simulink model "inverter_network"  (R2023a)
settings: Solver=ode4  StartTime=0.0  StopTime=0.8  FixedStep=1e-6  RelTol=1e-3
values from neighbouring files (symbols this model uses):
  C_gv = 1.5e-3    (= 0.0015)    [init.m]
  Cf = 2e-5    (= 2e-05)    [init.m]
  Cf_r = 1    [init.m]
  frequency = 50    [init.m]
  kpgi = 15    [init.m]
  kpi = 8    [init.m]
  kpv = 0.1    [init.m]
  krgi = 600    [init.m]
  krv = 100    [init.m]
  L_fv = 1.5e-3    (= 0.0015)    [init.m]
  L_line = 0.003*rbase/omega    (= 0.000152788745368)    [init.m]
  Lf = 4e-3    (= 0.004)    [init.m]
  Lf_r = 0.3    [init.m]
  Lg = 0.24e-3    (= 0.00024)    [init.m]
  omega = 2*pi*frequency    (= 314.159265359)    [init.m]
  R_line = 0.013*rbase    (= 0.208)    [init.m]
  vc_l = 0.03*rbase    (= 0.48)    [init.m]
  vdc = 400*1.88    (= 752)    [init.m]
  vref_rms = 300*(0.707*sqrt(3))    [init.m]
libraries: spsThreePhaseVIMeasurementLib x14, spsHalfBridgeConverterLib x9, spsThreePhaseSeriesRLCBranchLib x7, spsPower3phInstantaneousLib x6, spsThreePhaseParallelRLCBranchLib x5, spsabctoAlphaBetaZeroLib x5, spsGroundLib x4, spsAlphaBetaZerotoabcLib x3, spsDCVoltageSourceLib x3, eePwmGeneratorTwoLevel x3, spsPLL3phLib x2, spsdq0toAlphaBetaZeroLib x2
(part 1 of 2)
settings Model: Creator=MrSam  LastModifiedBy=15185

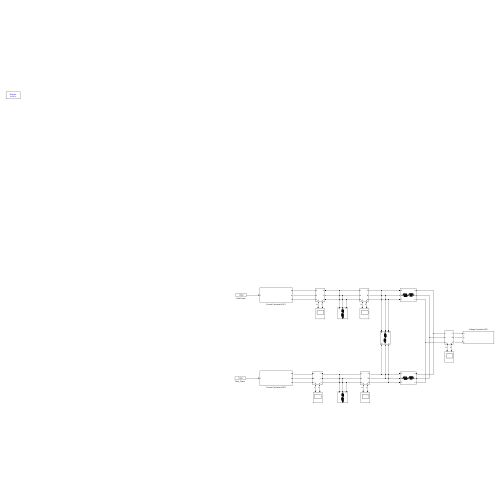
[thumbnail: Simulink's stored preview of the top-level diagram]
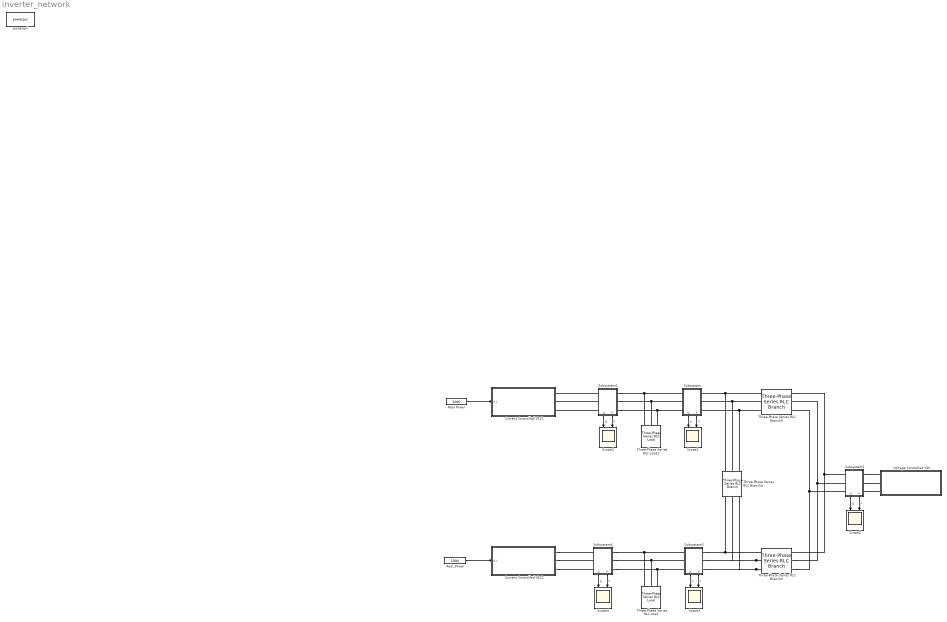
== system inverter_network ==
  Current Controlled VSC1 : Subsystem
  Current Controlled VSC2 : Subsystem
  Real Power : Constant  Value=1000
  Real_Power : Constant  Value=1000
  Scope{1..5} (5 alike) : Scope  NumInputPorts=2
  Subsystem : Subsystem
      settings: PortSchema="{\"entries\":[{\"content\":{\"sides\":[{\"content\":{\"connectorIds\":[\"LConn1\",\"LConn2\",\"LConn3\"]},\"type\":\"ConnectorPlacement.EquallySpacedRectSide\",\"uuid\":\"955e9456-33e7-4503-a1c1-a41c88bb3772\"},{\"content\":{\"connectorIds\":[\"RConn1\",\"RConn2\",\"RConn3\"],\"side\":\"RIGHT\"},\"type\":\"ConnectorPlacement.EquallySpacedRectSide\",\"uuid\":\"f38de2c4-935d-4540-b4e6-45221c91d1e6\"},{\"content\":{\"connectorIds\":[\"Out1\",\"Out2\"],\"side\":\"TOP\"},\"type\":\"ConnectorPlacement.EquallySpacedRectSide\",\"uuid\":\"a6953e65-ebf7-4510-908a-6e7d2a558034\"},{\"content\":{\"side\":\"BOTTOM\"},\"type\":\"ConnectorPlacement.EquallySpacedRectSide\",\"uuid\":\"e88c2e24-bb92-43a4-b254-c25644ec4733\"}]},\"type\":\"ConnectorPlacement.EquallySpacedConnector\",\"uuid\":\"5a2c0e39-8a05-4bc8-9b7c-68d8aae1862d\"}],\"packageUris\":[\"http://schema.mathworks.com/mf0/Connector/R2020b\"],\"version\":\"1.0\"}"
  Subsystem2 : Subsystem
      settings: PortSchema="{\"entries\":[{\"content\":{\"sides\":[{\"content\":{\"connectorIds\":[\"LConn1\",\"LConn2\",\"LConn3\"]},\"type\":\"ConnectorPlacement.EquallySpacedRectSide\",\"uuid\":\"955e9456-33e7-4503-a1c1-a41c88bb3772\"},{\"content\":{\"connectorIds\":[\"RConn1\",\"RConn2\",\"RConn3\"],\"side\":\"RIGHT\"},\"type\":\"ConnectorPlacement.EquallySpacedRectSide\",\"uuid\":\"f38de2c4-935d-4540-b4e6-45221c91d1e6\"},{\"content\":{\"side\":\"TOP\"},\"type\":\"ConnectorPlacement.EquallySpacedRectSide\",\"uuid\":\"a6953e65-ebf7-4510-908a-6e7d2a558034\"},{\"content\":{\"connectorIds\":[\"Out1\",\"Out2\"],\"side\":\"BOTTOM\"},\"type\":\"ConnectorPlacement.EquallySpacedRectSide\",\"uuid\":\"e88c2e24-bb92-43a4-b254-c25644ec4733\"}]},\"type\":\"ConnectorPlacement.EquallySpacedConnector\",\"uuid\":\"5a2c0e39-8a05-4bc8-9b7c-68d8aae1862d\"}],\"packageUris\":[\"http://schema.mathworks.com/mf0/Connector/R2020b\"],\"version\":\"1.0\"}"
  Subsystem3 : Subsystem
      settings: PortSchema="{\"entries\":[{\"content\":{\"sides\":[{\"content\":{\"connectorIds\":[\"LConn1\",\"LConn2\",\"LConn3\"]},\"type\":\"ConnectorPlacement.EquallySpacedRectSide\",\"uuid\":\"955e9456-33e7-4503-a1c1-a41c88bb3772\"},{\"content\":{\"connectorIds\":[\"RConn1\",\"RConn2\",\"RConn3\"],\"side\":\"RIGHT\"},\"type\":\"ConnectorPlacement.EquallySpacedRectSide\",\"uuid\":\"f38de2c4-935d-4540-b4e6-45221c91d1e6\"},{\"content\":{\"connectorIds\":[\"Out1\",\"Out2\"],\"side\":\"TOP\"},\"type\":\"ConnectorPlacement.EquallySpacedRectSide\",\"uuid\":\"a6953e65-ebf7-4510-908a-6e7d2a558034\"},{\"content\":{\"side\":\"BOTTOM\"},\"type\":\"ConnectorPlacement.EquallySpacedRectSide\",\"uuid\":\"e88c2e24-bb92-43a4-b254-c25644ec4733\"}]},\"type\":\"ConnectorPlacement.EquallySpacedConnector\",\"uuid\":\"5a2c0e39-8a05-4bc8-9b7c-68d8aae1862d\"}],\"packageUris\":[\"http://schema.mathworks.com/mf0/Connector/R2020b\"],\"version\":\"1.0\"}"
  Subsystem4 : Subsystem
      settings: PortSchema="{\"entries\":[{\"content\":{\"sides\":[{\"content\":{\"connectorIds\":[\"LConn1\",\"LConn2\",\"LConn3\"]},\"type\":\"ConnectorPlacement.EquallySpacedRectSide\",\"uuid\":\"955e9456-33e7-4503-a1c1-a41c88bb3772\"},{\"content\":{\"connectorIds\":[\"RConn1\",\"RConn2\",\"RConn3\"],\"side\":\"RIGHT\"},\"type\":\"ConnectorPlacement.EquallySpacedRectSide\",\"uuid\":\"f38de2c4-935d-4540-b4e6-45221c91d1e6\"},{\"content\":{\"side\":\"TOP\"},\"type\":\"ConnectorPlacement.EquallySpacedRectSide\",\"uuid\":\"a6953e65-ebf7-4510-908a-6e7d2a558034\"},{\"content\":{\"connectorIds\":[\"Out1\",\"Out2\"],\"side\":\"BOTTOM\"},\"type\":\"ConnectorPlacement.EquallySpacedRectSide\",\"uuid\":\"e88c2e24-bb92-43a4-b254-c25644ec4733\"}]},\"type\":\"ConnectorPlacement.EquallySpacedConnector\",\"uuid\":\"5a2c0e39-8a05-4bc8-9b7c-68d8aae1862d\"}],\"packageUris\":[\"http://schema.mathworks.com/mf0/Connector/R2020b\"],\"version\":\"1.0\"}"
  Subsystem5 : Subsystem
      settings: PortSchema="{\"entries\":[{\"content\":{\"sides\":[{\"content\":{\"connectorIds\":[\"LConn1\",\"LConn2\",\"LConn3\"]},\"type\":\"ConnectorPlacement.EquallySpacedRectSide\",\"uuid\":\"955e9456-33e7-4503-a1c1-a41c88bb3772\"},{\"content\":{\"connectorIds\":[\"RConn1\",\"RConn2\",\"RConn3\"],\"side\":\"RIGHT\"},\"type\":\"ConnectorPlacement.EquallySpacedRectSide\",\"uuid\":\"f38de2c4-935d-4540-b4e6-45221c91d1e6\"},{\"content\":{\"connectorIds\":[\"Out1\",\"Out2\"],\"side\":\"TOP\"},\"type\":\"ConnectorPlacement.EquallySpacedRectSide\",\"uuid\":\"a6953e65-ebf7-4510-908a-6e7d2a558034\"},{\"content\":{\"side\":\"BOTTOM\"},\"type\":\"ConnectorPlacement.EquallySpacedRectSide\",\"uuid\":\"e88c2e24-bb92-43a4-b254-c25644ec4733\"}]},\"type\":\"ConnectorPlacement.EquallySpacedConnector\",\"uuid\":\"5a2c0e39-8a05-4bc8-9b7c-68d8aae1862d\"}],\"packageUris\":[\"http://schema.mathworks.com/mf0/Connector/R2020b\"],\"version\":\"1.0\"}"
  Three-Phase Series RLC Branch4 : spsThreePhaseSeriesRLCBranchLib/Three-Phase Series RLC Branch  LConnTagsString=A|B|C  RConnTagsString=A|B|C  BranchType=RL  Resistance=R_line  Inductance=L_line  Capacitance=0  Measurements=None
  Three-Phase Series RLC Branch5 : spsThreePhaseSeriesRLCBranchLib/Three-Phase Series RLC Branch  LConnTagsString=A|B|C  RConnTagsString=A|B|C  BranchType=RL  Resistance=R_line  Inductance=L_line  Capacitance=0  Measurements=None
  Three-Phase Series RLC Branch6 : spsThreePhaseSeriesRLCBranchLib/Three-Phase Series RLC Branch  LConnTagsString=A|B|C  RConnTagsString=A|B|C  BranchType=RL  Resistance=R_line  Inductance=L_line  Capacitance=0  Measurements=None
  Three-Phase Series RLC Load : spsThreePhaseSeriesRLCLoadLib/Three-Phase Series RLC Load  LConnTagsString=A|B|C  Configuration=Y (grounded)  NominalVoltage=367  Vabc=[1e3 1e3 1e3]  Vabcp=[1e3 1e3 1e3]  NominalFrequency=frequency  UnbalancedPower=off  ActivePower=1500  InductivePower=500  CapacitivePower=0  Pabc=[10e3 9e3 11e3]  QLabc=[100 90 110]  QCabc=[100 90 110]  Pabcp=[10e3 9e3 11e3]  QLabcp=[100 90 110]  QCabcp=[100 90 110]  Measurements=None  LoadType=constant Z
  Three-Phase Series RLC Load1 : spsThreePhaseSeriesRLCLoadLib/Three-Phase Series RLC Load  LConnTagsString=A|B|C  Configuration=Y (grounded)  NominalVoltage=367  Vabc=[1e3 1e3 1e3]  Vabcp=[1e3 1e3 1e3]  NominalFrequency=frequency  UnbalancedPower=off  ActivePower=1500  InductivePower=500  CapacitivePower=0  Pabc=[10e3 9e3 11e3]  QLabc=[100 90 110]  QCabc=[100 90 110]  Pabcp=[10e3 9e3 11e3]  QLabcp=[100 90 110]  QCabcp=[100 90 110]  Measurements=None  LoadType=constant Z
  Voltage Controlled VSC : Subsystem
  powergui : spspowerguiLib/powergui  Priority=1  SimulationMode=Discrete  SampleTime=1e-6  frequency=60  Iterations=50  frequencyindice=50  Pbase=100e6  ErrMax=1e-4  UnitsV=kV  UnitsW=MW  buscounter=0  FunctionMessages=off  echomessages=off  EnableUseOfTLC=off  CurrentSourceSwitches=off  DisableSnubberDevices=off  DisableRonSwitches=off  DisableVfSwitches=off  DisplayEquations=off  AutomaticDiscreteSolvers=off  SolverType=Tustin/Backward Euler (TBE)  Interpol=off  ExternalGateDelay=off  methode=off  Ts=100  x0status=blocks  SPID=on  SwTol=0  HookPort=off  NonlinearTolerance=1e-4  nMaxIteration=100  ContinueOnMaxIteration=off  RestoreLinks=warning  ResistiveCurrentMeasurement=off  Frange=[0:2:500]  Ylog=off  Xlog=on  ShowGrid=off  save=off  variable=ZData  structure=0  ZoomFFT=off  StartTime=0.0  cycles=1  DisplayStyle=1  fundamental=60  FreqAxis=off  MaxFrequency=1000  frequencyindicesteady=1  RmsSteady=1  display=off
  wires:
  Real Power/1 -> Current Controlled VSC1/1(In1)
  Real_Power/1 -> Current Controlled VSC2/1(In1)
  Subsystem/1(P) -> Scope1/2  "P"
  Subsystem/2(Q) -> Scope1/1  "Q"
  Subsystem2/1(Q) -> Scope2/1  "Q"
  Subsystem2/2(P) -> Scope2/2  "P"
  Subsystem3/2(Q) -> Scope3/1  "Q"
  Subsystem3/1(P) -> Scope3/2  "P"
  Subsystem4/2(P) -> Scope4/2  "P"
  Subsystem4/1(Q) -> Scope4/1  "Q"
  Subsystem5/1(P) -> Scope5/2  "P"
  Subsystem5/2(Q) -> Scope5/1  "Q"
  connections:
  Three-Phase Series RLC Branch6/LConn3 -- Subsystem3/LConn1 -- Three-Phase Series RLC Branch4/RConn3
  Three-Phase Series RLC Load/LConn3 -- Subsystem4/RConn3 -- Subsystem3/RConn1
  Three-Phase Series RLC Load/LConn2 -- Subsystem4/RConn2 -- Subsystem3/RConn2
  Three-Phase Series RLC Load/LConn1 -- Subsystem4/RConn1 -- Subsystem3/RConn3
  Three-Phase Series RLC Load1/LConn3 -- Subsystem2/RConn3 -- Subsystem/RConn1
  Three-Phase Series RLC Branch5/LConn1 -- Three-Phase Series RLC Branch4/LConn1 -- Subsystem/LConn3
  Three-Phase Series RLC Branch5/LConn2 -- Three-Phase Series RLC Branch4/LConn2 -- Subsystem/LConn2
  Three-Phase Series RLC Branch5/LConn3 -- Three-Phase Series RLC Branch4/LConn3 -- Subsystem/LConn1
  Three-Phase Series RLC Branch4/RConn1 -- Subsystem3/LConn3 -- Three-Phase Series RLC Branch6/LConn1
  Three-Phase Series RLC Branch6/LConn2 -- Subsystem3/LConn2 -- Three-Phase Series RLC Branch4/RConn2
  Subsystem5/LConn1 -- Voltage Controlled VSC/RConn3
  Subsystem5/LConn2 -- Voltage Controlled VSC/RConn2
  Three-Phase Series RLC Branch5/RConn1 -- Subsystem5/RConn3 -- Three-Phase Series RLC Branch6/RConn1
  Three-Phase Series RLC Load1/LConn2 -- Subsystem2/RConn2 -- Subsystem/RConn2
  Three-Phase Series RLC Load1/LConn1 -- Subsystem2/RConn1 -- Subsystem/RConn3
  Subsystem2/LConn2 -- Current Controlled VSC1/RConn2
  Subsystem2/LConn1 -- Current Controlled VSC1/RConn1
  Subsystem2/LConn3 -- Current Controlled VSC1/RConn3
  Current Controlled VSC2/RConn3 -- Subsystem4/LConn3
  Current Controlled VSC2/RConn2 -- Subsystem4/LConn2
  Current Controlled VSC2/RConn1 -- Subsystem4/LConn1
  Subsystem5/LConn3 -- Voltage Controlled VSC/RConn1
  Three-Phase Series RLC Branch6/RConn2 -- Subsystem5/RConn2 -- Three-Phase Series RLC Branch5/RConn2
  Three-Phase Series RLC Branch6/RConn3 -- Subsystem5/RConn1 -- Three-Phase Series RLC Branch5/RConn3

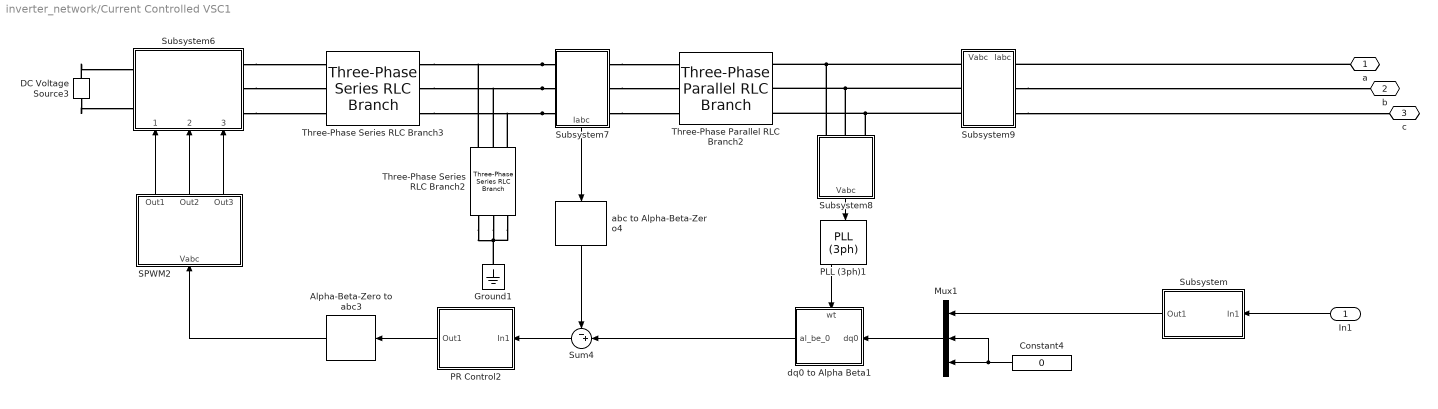
== system inverter_network/Current Controlled VSC1 ==
  In1 : Inport
  Alpha-Beta-Zero to abc3 : spsAlphaBetaZerotoabcLib/Alpha-Beta-Zero to abc
      settings: LibrarySourceBlock=|
      | sps_lib/Control/Alpha-Beta-Zero
      | to abc
  Constant4 : Constant  Value=0
  DC Voltage Source3 : spsDCVoltageSourceLib/DC Voltage Source  Amplitude=600  Measurements=None
  Ground1 : spsGroundLib/Ground  LConnTagsString=a
  Mux1 : Mux  Inputs=3
  PLL (3ph)1 : spsPLL3phLib/PLL (3ph)  Fmin=45  Par_Init=[0, frequency]  ParK=[180, 3200, 1]  TcD=1e-4  MaxRateChangeFreq=12  FilterCutOffFreq=25  Ts=0  AGC=on
  PR Control2 : Subsystem
  SPWM2 : Subsystem
  Subsystem : Subsystem
  Subsystem6 : Subsystem
      settings: PortSchema="{\"entries\":[{\"content\":{\"sides\":[{\"content\":{\"connectorIds\":[\"LConn1\",\"LConn2\"]},\"type\":\"ConnectorPlacement.EquallySpacedRectSide\",\"uuid\":\"21765539-0567-4900-b052-fb0c809e49e6\"},{\"content\":{\"connectorIds\":[\"RConn1\",\"RConn2\",\"RConn3\"],\"side\":\"RIGHT\"},\"type\":\"ConnectorPlacement.EquallySpacedRectSide\",\"uuid\":\"da60e673-aefd-4ef6-b5b1-e42a137712f7\"},{\"content\":{\"side\":\"TOP\"},\"type\":\"ConnectorPlacement.EquallySpacedRectSide\",\"uuid\":\"b6e664be-1a8c-4c9c-bd73-b93bd6e53381\"},{\"content\":{\"connectorIds\":[\"In1\",\"In2\",\"In3\"],\"side\":\"BOTTOM\"},\"type\":\"ConnectorPlacement.EquallySpacedRectSide\",\"uuid\":\"f785bed7-33ce-41e0-9620-ddd9724794f7\"}]},\"type\":\"ConnectorPlacement.EquallySpacedConnector\",\"uuid\":\"3eaff965-cae1-44ee-8f3f-ae8df46f200b\"}],\"packageUris\":[\"http://schema.mathworks.com/mf0/Connector/R2020b\"],\"version\":\"1.0\"}"
  Subsystem7 : Subsystem
      settings: PortSchema="{\"entries\":[{\"content\":{\"sides\":[{\"content\":{\"connectorIds\":[\"LConn1\",\"LConn2\",\"LConn3\"]},\"type\":\"ConnectorPlacement.EquallySpacedRectSide\",\"uuid\":\"5e649b81-8d67-47fb-b51d-7fa1d294a0fa\"},{\"content\":{\"connectorIds\":[\"RConn1\",\"RConn2\",\"RConn3\"],\"side\":\"RIGHT\"},\"type\":\"ConnectorPlacement.EquallySpacedRectSide\",\"uuid\":\"b8ce6232-1e24-4620-bb1d-7a04b9b53c9d\"},{\"content\":{\"side\":\"TOP\"},\"type\":\"ConnectorPlacement.EquallySpacedRectSide\",\"uuid\":\"aabe5581-fbc6-4714-8701-49215a0525de\"},{\"content\":{\"connectorIds\":[\"Out1\"],\"side\":\"BOTTOM\"},\"type\":\"ConnectorPlacement.EquallySpacedRectSide\",\"uuid\":\"d004e6ed-4fae-491a-82a2-0495bcb0f8c1\"}]},\"type\":\"ConnectorPlacement.EquallySpacedConnector\",\"uuid\":\"9c494b08-2ee2-4375-b64d-9899f5cce3ba\"}],\"packageUris\":[\"http://schema.mathworks.com/mf0/Connector/R2020b\"],\"version\":\"1.0\"}"
  Subsystem8 : Subsystem
  Subsystem9 : Subsystem
      settings: PortSchema="{\"entries\":[{\"content\":{\"sides\":[{\"content\":{\"connectorIds\":[\"LConn1\",\"LConn2\",\"LConn3\"]},\"type\":\"ConnectorPlacement.EquallySpacedRectSide\",\"uuid\":\"5e649b81-8d67-47fb-b51d-7fa1d294a0fa\"},{\"content\":{\"connectorIds\":[\"RConn1\",\"RConn2\",\"RConn3\"],\"side\":\"RIGHT\"},\"type\":\"ConnectorPlacement.EquallySpacedRectSide\",\"uuid\":\"b8ce6232-1e24-4620-bb1d-7a04b9b53c9d\"},{\"content\":{\"connectorIds\":[\"Out1\",\"Out2\"],\"side\":\"TOP\"},\"type\":\"ConnectorPlacement.EquallySpacedRectSide\",\"uuid\":\"aabe5581-fbc6-4714-8701-49215a0525de\"}]},\"type\":\"ConnectorPlacement.EquallySpacedConnector\",\"uuid\":\"9c494b08-2ee2-4375-b64d-9899f5cce3ba\"}],\"packageUris\":[\"http://schema.mathworks.com/mf0/Connector/R2020b\"],\"version\":\"1.0\"}"
  Sum4 : Sum  Inputs=-+|
  Three-Phase Parallel RLC Branch2 : spsThreePhaseParallelRLCBranchLib/Three-Phase Parallel RLC Branch  LConnTagsString=A|B|C  RConnTagsString=A|B|C  BranchType=L  Resistance=1  Inductance=Lg  Capacitance=1e-6  Measurements=None
  Three-Phase Series RLC Branch2 : spsThreePhaseSeriesRLCBranchLib/Three-Phase Series RLC Branch  LConnTagsString=A|B|C  RConnTagsString=A|B|C  BranchType=RC  Resistance=Cf_r  Inductance=1e-3  Capacitance=Cf  Measurements=None
  Three-Phase Series RLC Branch3 : spsThreePhaseSeriesRLCBranchLib/Three-Phase Series RLC Branch  LConnTagsString=A|B|C  RConnTagsString=A|B|C  BranchType=RL  Resistance=Lf_r  Inductance=Lf  Capacitance=1e-6  Measurements=None
  abc to Alpha-Beta-Zero4 : spsabctoAlphaBetaZeroLib/abc to Alpha-Beta-Zero
  dq0 to Alpha Beta1 : Subsystem
      settings: PortSchema="{\"entries\":[{\"content\":{\"sides\":[{\"content\":{\"connectorIds\":[\"In1\"]},\"type\":\"ConnectorPlacement.EquallySpacedRectSide\",\"uuid\":\"2957cf7a-c1c3-4848-9407-b6952c647f30\"},{\"content\":{\"connectorIds\":[\"Out1\"],\"side\":\"RIGHT\"},\"type\":\"ConnectorPlacement.EquallySpacedRectSide\",\"uuid\":\"7a8beffb-254d-479d-a697-96ba44ae1442\"},{\"content\":{\"connectorIds\":[\"In2\"],\"side\":\"TOP\"},\"type\":\"ConnectorPlacement.EquallySpacedRectSide\",\"uuid\":\"8b95608f-2c8d-45bf-9e71-a12dce74a0a0\"}]},\"type\":\"ConnectorPlacement.EquallySpacedConnector\",\"uuid\":\"69f38502-e33d-4dbf-872c-0372c4b36551\"}],\"packageUris\":[\"http://schema.mathworks.com/mf0/Connector/R2020b\"],\"version\":\"1.0\"}"
  a : PMIOPort  Side=Right
  b : PMIOPort  Port=2  Side=Right
  c : PMIOPort  Port=3  Side=Right
  wires:
  Subsystem8/1(Vabc) -> PLL (3ph)1/1
  PR Control2/1(Out1) -> Alpha-Beta-Zero to abc3/1
  PLL (3ph)1/2 -> dq0 to Alpha Beta1/2(wt)
  Subsystem7/1(Iabc) -> abc to Alpha-Beta-Zero4/1
  Constant4/1 -> Mux1/2, Mux1/3
  abc to Alpha-Beta-Zero4/1 -> Sum4/1
  SPWM2/2(Out2) -> Subsystem6/2("  2")
  Alpha-Beta-Zero to abc3/1 -> SPWM2/1(Vabc)
  SPWM2/1(Out1) -> Subsystem6/1(" 1 ")
  Sum4/1 -> PR Control2/1(In1)
  dq0 to Alpha Beta1/1(al_be_0) -> Sum4/2
  SPWM2/3(Out3) -> Subsystem6/3("  3")
  Mux1/1 -> dq0 to Alpha Beta1/1(dq0)
  In1/1 -> Subsystem/1(In1)
  Subsystem/1(Out1) -> Mux1/1
  connections:
  Subsystem7/RConn3 -- Three-Phase Parallel RLC Branch2/LConn3
  Subsystem9/LConn3 -- Subsystem8/LConn3 -- Three-Phase Parallel RLC Branch2/RConn3
  Subsystem7/LConn1 -- Three-Phase Series RLC Branch2/LConn1 -- Three-Phase Series RLC Branch3/RConn1
  Subsystem6/RConn3 -- Three-Phase Series RLC Branch3/LConn3
  a/RConn1 -- Subsystem9/RConn1
  Subsystem9/LConn1 -- Subsystem8/LConn1 -- Three-Phase Parallel RLC Branch2/RConn1
  DC Voltage Source3/RConn1 -- Subsystem6/LConn1
  Subsystem9/LConn2 -- Subsystem8/LConn2 -- Three-Phase Parallel RLC Branch2/RConn2
  DC Voltage Source3/LConn1 -- Subsystem6/LConn2
  Three-Phase Series RLC Branch2/RConn2 -- Ground1/LConn1 -- Three-Phase Series RLC Branch2/RConn3 -- Three-Phase Series RLC Branch2/RConn1
  Subsystem7/LConn3 -- Three-Phase Series RLC Branch2/LConn3 -- Three-Phase Series RLC Branch3/RConn3
  Subsystem6/RConn1 -- Three-Phase Series RLC Branch3/LConn1
  Subsystem7/RConn1 -- Three-Phase Parallel RLC Branch2/LConn1
  Subsystem7/LConn2 -- Three-Phase Series RLC Branch2/LConn2 -- Three-Phase Series RLC Branch3/RConn2
  Subsystem6/RConn2 -- Three-Phase Series RLC Branch3/LConn2
  Subsystem9/RConn2 -- b/RConn1
  Subsystem7/RConn2 -- Three-Phase Parallel RLC Branch2/LConn2
  Subsystem9/RConn3 -- c/RConn1

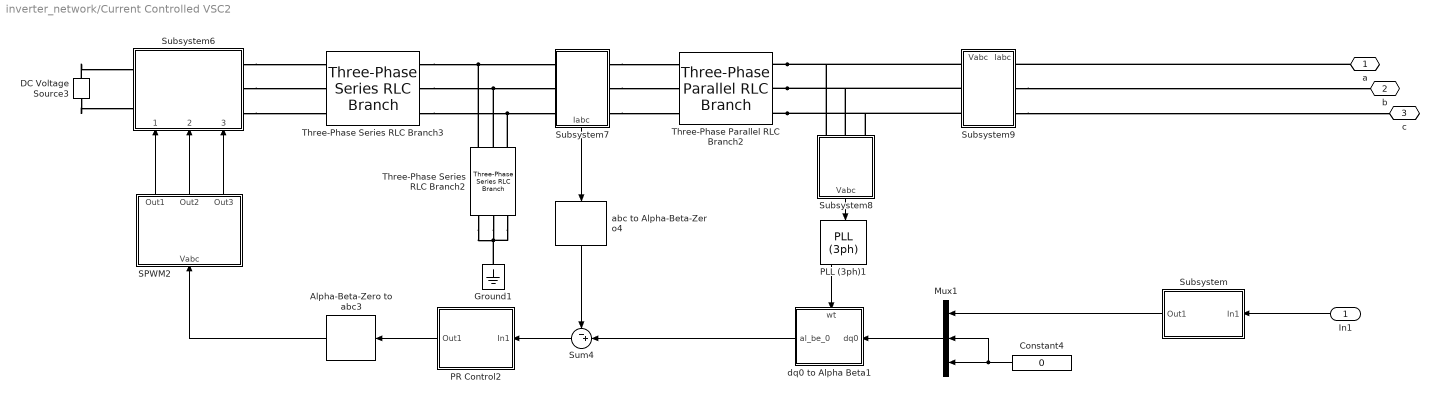
== system inverter_network/Current Controlled VSC2 ==
  In1 : Inport
  Alpha-Beta-Zero to abc3 : spsAlphaBetaZerotoabcLib/Alpha-Beta-Zero to abc
      settings: LibrarySourceBlock=|
      | sps_lib/Control/Alpha-Beta-Zero
      | to abc
  Constant4 : Constant  Value=0
  DC Voltage Source3 : spsDCVoltageSourceLib/DC Voltage Source  Amplitude=600  Measurements=None
  Ground1 : spsGroundLib/Ground  LConnTagsString=a
  Mux1 : Mux  Inputs=3
  PLL (3ph)1 : spsPLL3phLib/PLL (3ph)  Fmin=45  Par_Init=[0, frequency]  ParK=[180, 3200, 1]  TcD=1e-4  MaxRateChangeFreq=12  FilterCutOffFreq=25  Ts=0  AGC=on
  PR Control2 : Subsystem
  SPWM2 : Subsystem
  Subsystem : Subsystem
  Subsystem6 : Subsystem
      settings: PortSchema="{\"entries\":[{\"content\":{\"sides\":[{\"content\":{\"connectorIds\":[\"LConn1\",\"LConn2\"]},\"type\":\"ConnectorPlacement.EquallySpacedRectSide\",\"uuid\":\"21765539-0567-4900-b052-fb0c809e49e6\"},{\"content\":{\"connectorIds\":[\"RConn1\",\"RConn2\",\"RConn3\"],\"side\":\"RIGHT\"},\"type\":\"ConnectorPlacement.EquallySpacedRectSide\",\"uuid\":\"da60e673-aefd-4ef6-b5b1-e42a137712f7\"},{\"content\":{\"side\":\"TOP\"},\"type\":\"ConnectorPlacement.EquallySpacedRectSide\",\"uuid\":\"b6e664be-1a8c-4c9c-bd73-b93bd6e53381\"},{\"content\":{\"connectorIds\":[\"In1\",\"In2\",\"In3\"],\"side\":\"BOTTOM\"},\"type\":\"ConnectorPlacement.EquallySpacedRectSide\",\"uuid\":\"f785bed7-33ce-41e0-9620-ddd9724794f7\"}]},\"type\":\"ConnectorPlacement.EquallySpacedConnector\",\"uuid\":\"3eaff965-cae1-44ee-8f3f-ae8df46f200b\"}],\"packageUris\":[\"http://schema.mathworks.com/mf0/Connector/R2020b\"],\"version\":\"1.0\"}"
  Subsystem7 : Subsystem
      settings: PortSchema="{\"entries\":[{\"content\":{\"sides\":[{\"content\":{\"connectorIds\":[\"LConn1\",\"LConn2\",\"LConn3\"]},\"type\":\"ConnectorPlacement.EquallySpacedRectSide\",\"uuid\":\"5e649b81-8d67-47fb-b51d-7fa1d294a0fa\"},{\"content\":{\"connectorIds\":[\"RConn1\",\"RConn2\",\"RConn3\"],\"side\":\"RIGHT\"},\"type\":\"ConnectorPlacement.EquallySpacedRectSide\",\"uuid\":\"b8ce6232-1e24-4620-bb1d-7a04b9b53c9d\"},{\"content\":{\"side\":\"TOP\"},\"type\":\"ConnectorPlacement.EquallySpacedRectSide\",\"uuid\":\"aabe5581-fbc6-4714-8701-49215a0525de\"},{\"content\":{\"connectorIds\":[\"Out1\"],\"side\":\"BOTTOM\"},\"type\":\"ConnectorPlacement.EquallySpacedRectSide\",\"uuid\":\"d004e6ed-4fae-491a-82a2-0495bcb0f8c1\"}]},\"type\":\"ConnectorPlacement.EquallySpacedConnector\",\"uuid\":\"9c494b08-2ee2-4375-b64d-9899f5cce3ba\"}],\"packageUris\":[\"http://schema.mathworks.com/mf0/Connector/R2020b\"],\"version\":\"1.0\"}"
  Subsystem8 : Subsystem
  Subsystem9 : Subsystem
      settings: PortSchema="{\"entries\":[{\"content\":{\"sides\":[{\"content\":{\"connectorIds\":[\"LConn1\",\"LConn2\",\"LConn3\"]},\"type\":\"ConnectorPlacement.EquallySpacedRectSide\",\"uuid\":\"5e649b81-8d67-47fb-b51d-7fa1d294a0fa\"},{\"content\":{\"connectorIds\":[\"RConn1\",\"RConn2\",\"RConn3\"],\"side\":\"RIGHT\"},\"type\":\"ConnectorPlacement.EquallySpacedRectSide\",\"uuid\":\"b8ce6232-1e24-4620-bb1d-7a04b9b53c9d\"},{\"content\":{\"connectorIds\":[\"Out1\",\"Out2\"],\"side\":\"TOP\"},\"type\":\"ConnectorPlacement.EquallySpacedRectSide\",\"uuid\":\"aabe5581-fbc6-4714-8701-49215a0525de\"}]},\"type\":\"ConnectorPlacement.EquallySpacedConnector\",\"uuid\":\"9c494b08-2ee2-4375-b64d-9899f5cce3ba\"}],\"packageUris\":[\"http://schema.mathworks.com/mf0/Connector/R2020b\"],\"version\":\"1.0\"}"
  Sum4 : Sum  Inputs=-+|
  Three-Phase Parallel RLC Branch2 : spsThreePhaseParallelRLCBranchLib/Three-Phase Parallel RLC Branch  LConnTagsString=A|B|C  RConnTagsString=A|B|C  BranchType=L  Resistance=1  Inductance=Lg  Capacitance=1e-6  Measurements=None
  Three-Phase Series RLC Branch2 : spsThreePhaseSeriesRLCBranchLib/Three-Phase Series RLC Branch  LConnTagsString=A|B|C  RConnTagsString=A|B|C  BranchType=RC  Resistance=Cf_r  Inductance=1e-3  Capacitance=Cf  Measurements=None
  Three-Phase Series RLC Branch3 : spsThreePhaseSeriesRLCBranchLib/Three-Phase Series RLC Branch  LConnTagsString=A|B|C  RConnTagsString=A|B|C  BranchType=RL  Resistance=Lf_r  Inductance=Lf  Capacitance=1e-6  Measurements=None
  abc to Alpha-Beta-Zero4 : spsabctoAlphaBetaZeroLib/abc to Alpha-Beta-Zero
  dq0 to Alpha Beta1 : Subsystem
      settings: PortSchema="{\"entries\":[{\"content\":{\"sides\":[{\"content\":{\"connectorIds\":[\"In1\"]},\"type\":\"ConnectorPlacement.EquallySpacedRectSide\",\"uuid\":\"2957cf7a-c1c3-4848-9407-b6952c647f30\"},{\"content\":{\"connectorIds\":[\"Out1\"],\"side\":\"RIGHT\"},\"type\":\"ConnectorPlacement.EquallySpacedRectSide\",\"uuid\":\"7a8beffb-254d-479d-a697-96ba44ae1442\"},{\"content\":{\"connectorIds\":[\"In2\"],\"side\":\"TOP\"},\"type\":\"ConnectorPlacement.EquallySpacedRectSide\",\"uuid\":\"8b95608f-2c8d-45bf-9e71-a12dce74a0a0\"}]},\"type\":\"ConnectorPlacement.EquallySpacedConnector\",\"uuid\":\"69f38502-e33d-4dbf-872c-0372c4b36551\"}],\"packageUris\":[\"http://schema.mathworks.com/mf0/Connector/R2020b\"],\"version\":\"1.0\"}"
  a : PMIOPort  Side=Right
  b : PMIOPort  Port=2  Side=Right
  c : PMIOPort  Port=3  Side=Right
  wires:
  Subsystem8/1(Vabc) -> PLL (3ph)1/1
  PR Control2/1(Out1) -> Alpha-Beta-Zero to abc3/1
  PLL (3ph)1/2 -> dq0 to Alpha Beta1/2(wt)
  Subsystem7/1(Iabc) -> abc to Alpha-Beta-Zero4/1
  Constant4/1 -> Mux1/2, Mux1/3
  abc to Alpha-Beta-Zero4/1 -> Sum4/1
  SPWM2/2(Out2) -> Subsystem6/2("  2")
  Alpha-Beta-Zero to abc3/1 -> SPWM2/1(Vabc)
  SPWM2/1(Out1) -> Subsystem6/1(" 1 ")
  Sum4/1 -> PR Control2/1(In1)
  dq0 to Alpha Beta1/1(al_be_0) -> Sum4/2
  SPWM2/3(Out3) -> Subsystem6/3("  3")
  Mux1/1 -> dq0 to Alpha Beta1/1(dq0)
  In1/1 -> Subsystem/1(In1)
  Subsystem/1(Out1) -> Mux1/1
  connections:
  Subsystem7/RConn3 -- Three-Phase Parallel RLC Branch2/LConn3
  Three-Phase Parallel RLC Branch2/RConn3 -- Subsystem9/LConn3 -- Subsystem8/LConn3
  Three-Phase Series RLC Branch3/RConn1 -- Subsystem7/LConn1 -- Three-Phase Series RLC Branch2/LConn1
  Subsystem6/RConn3 -- Three-Phase Series RLC Branch3/LConn3
  a/RConn1 -- Subsystem9/RConn1
  Three-Phase Parallel RLC Branch2/RConn1 -- Subsystem9/LConn1 -- Subsystem8/LConn1
  DC Voltage Source3/RConn1 -- Subsystem6/LConn1
  Three-Phase Parallel RLC Branch2/RConn2 -- Subsystem9/LConn2 -- Subsystem8/LConn2
  DC Voltage Source3/LConn1 -- Subsystem6/LConn2
  Three-Phase Series RLC Branch2/RConn3 -- Three-Phase Series RLC Branch2/RConn1 -- Three-Phase Series RLC Branch2/RConn2 -- Ground1/LConn1
  Three-Phase Series RLC Branch3/RConn3 -- Subsystem7/LConn3 -- Three-Phase Series RLC Branch2/LConn3
  Subsystem6/RConn1 -- Three-Phase Series RLC Branch3/LConn1
  Subsystem7/RConn1 -- Three-Phase Parallel RLC Branch2/LConn1
  Three-Phase Series RLC Branch3/RConn2 -- Subsystem7/LConn2 -- Three-Phase Series RLC Branch2/LConn2
  Subsystem6/RConn2 -- Three-Phase Series RLC Branch3/LConn2
  Subsystem9/RConn2 -- b/RConn1
  Subsystem7/RConn2 -- Three-Phase Parallel RLC Branch2/LConn2
  Subsystem9/RConn3 -- c/RConn1

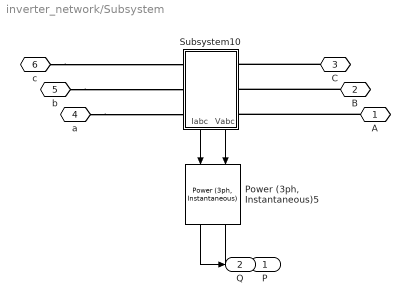
== system inverter_network/Subsystem ==
  "Power (3ph, Instantaneous)5" : spsPower3phInstantaneousLib/Power (3ph, Instantaneous)
  Subsystem10 : Subsystem
      settings: PortSchema="{\"entries\":[{\"content\":{\"sides\":[{\"content\":{\"connectorIds\":[\"LConn1\",\"LConn2\",\"LConn3\"]},\"type\":\"ConnectorPlacement.EquallySpacedRectSide\",\"uuid\":\"5e649b81-8d67-47fb-b51d-7fa1d294a0fa\"},{\"content\":{\"connectorIds\":[\"RConn1\",\"RConn2\",\"RConn3\"],\"side\":\"RIGHT\"},\"type\":\"ConnectorPlacement.EquallySpacedRectSide\",\"uuid\":\"b8ce6232-1e24-4620-bb1d-7a04b9b53c9d\"},{\"content\":{\"connectorIds\":[\"Out1\",\"Out2\"],\"side\":\"TOP\"},\"type\":\"ConnectorPlacement.EquallySpacedRectSide\",\"uuid\":\"aabe5581-fbc6-4714-8701-49215a0525de\"}]},\"type\":\"ConnectorPlacement.EquallySpacedConnector\",\"uuid\":\"9c494b08-2ee2-4375-b64d-9899f5cce3ba\"}],\"packageUris\":[\"http://schema.mathworks.com/mf0/Connector/R2020b\"],\"version\":\"1.0\"}"
  A : PMIOPort  Side=Left
  B : PMIOPort  Port=2  Side=Left
  C : PMIOPort  Port=3  Side=Left
  a : PMIOPort  Port=4  Side=Right
  b : PMIOPort  Port=5  Side=Right
  c : PMIOPort  Port=6  Side=Right
  P : Outport
  Q : Outport  Port=2
  wires:
  Subsystem10/1(Vabc) -> "Power (3ph, Instantaneous)5"/1
  Subsystem10/2(Iabc) -> "Power (3ph, Instantaneous)5"/2
  "Power (3ph, Instantaneous)5"/2 -> Q/1
  "Power (3ph, Instantaneous)5"/1 -> P/1
  connections:
  C/RConn1 -- Subsystem10/LConn3
  c/RConn1 -- Subsystem10/RConn3
  a/RConn1 -- Subsystem10/RConn1
  b/RConn1 -- Subsystem10/RConn2
  B/RConn1 -- Subsystem10/LConn2
  A/RConn1 -- Subsystem10/LConn1

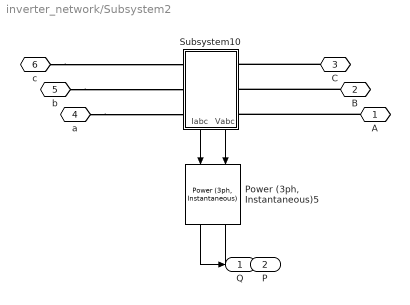
== system inverter_network/Subsystem2 ==
  "Power (3ph, Instantaneous)5" : spsPower3phInstantaneousLib/Power (3ph, Instantaneous)
  Subsystem10 : Subsystem
      settings: PortSchema="{\"entries\":[{\"content\":{\"sides\":[{\"content\":{\"connectorIds\":[\"LConn1\",\"LConn2\",\"LConn3\"]},\"type\":\"ConnectorPlacement.EquallySpacedRectSide\",\"uuid\":\"5e649b81-8d67-47fb-b51d-7fa1d294a0fa\"},{\"content\":{\"connectorIds\":[\"RConn1\",\"RConn2\",\"RConn3\"],\"side\":\"RIGHT\"},\"type\":\"ConnectorPlacement.EquallySpacedRectSide\",\"uuid\":\"b8ce6232-1e24-4620-bb1d-7a04b9b53c9d\"},{\"content\":{\"connectorIds\":[\"Out1\",\"Out2\"],\"side\":\"TOP\"},\"type\":\"ConnectorPlacement.EquallySpacedRectSide\",\"uuid\":\"aabe5581-fbc6-4714-8701-49215a0525de\"}]},\"type\":\"ConnectorPlacement.EquallySpacedConnector\",\"uuid\":\"9c494b08-2ee2-4375-b64d-9899f5cce3ba\"}],\"packageUris\":[\"http://schema.mathworks.com/mf0/Connector/R2020b\"],\"version\":\"1.0\"}"
  A : PMIOPort  Side=Left
  B : PMIOPort  Port=2  Side=Left
  C : PMIOPort  Port=3  Side=Left
  a : PMIOPort  Port=4  Side=Right
  b : PMIOPort  Port=5  Side=Right
  c : PMIOPort  Port=6  Side=Right
  Q : Outport
  P : Outport  Port=2
  wires:
  Subsystem10/1(Vabc) -> "Power (3ph, Instantaneous)5"/1
  Subsystem10/2(Iabc) -> "Power (3ph, Instantaneous)5"/2
  "Power (3ph, Instantaneous)5"/2 -> Q/1
  "Power (3ph, Instantaneous)5"/1 -> P/1
  connections:
  C/RConn1 -- Subsystem10/LConn3
  c/RConn1 -- Subsystem10/RConn3
  a/RConn1 -- Subsystem10/RConn1
  b/RConn1 -- Subsystem10/RConn2
  B/RConn1 -- Subsystem10/LConn2
  A/RConn1 -- Subsystem10/LConn1

== system inverter_network/Subsystem3 ==
  "Power (3ph, Instantaneous)5" : spsPower3phInstantaneousLib/Power (3ph, Instantaneous)
  Subsystem10 : Subsystem
      settings: PortSchema="{\"entries\":[{\"content\":{\"sides\":[{\"content\":{\"connectorIds\":[\"LConn1\",\"LConn2\",\"LConn3\"]},\"type\":\"ConnectorPlacement.EquallySpacedRectSide\",\"uuid\":\"5e649b81-8d67-47fb-b51d-7fa1d294a0fa\"},{\"content\":{\"connectorIds\":[\"RConn1\",\"RConn2\",\"RConn3\"],\"side\":\"RIGHT\"},\"type\":\"ConnectorPlacement.EquallySpacedRectSide\",\"uuid\":\"b8ce6232-1e24-4620-bb1d-7a04b9b53c9d\"},{\"content\":{\"connectorIds\":[\"Out1\",\"Out2\"],\"side\":\"TOP\"},\"type\":\"ConnectorPlacement.EquallySpacedRectSide\",\"uuid\":\"aabe5581-fbc6-4714-8701-49215a0525de\"}]},\"type\":\"ConnectorPlacement.EquallySpacedConnector\",\"uuid\":\"9c494b08-2ee2-4375-b64d-9899f5cce3ba\"}],\"packageUris\":[\"http://schema.mathworks.com/mf0/Connector/R2020b\"],\"version\":\"1.0\"}"
  A : PMIOPort  Side=Left
  B : PMIOPort  Port=2  Side=Left
  C : PMIOPort  Port=3  Side=Left
  a : PMIOPort  Port=4  Side=Right
  b : PMIOPort  Port=5  Side=Right
  c : PMIOPort  Port=6  Side=Right
  P : Outport
  Q : Outport  Port=2
  wires:
  Subsystem10/1(Vabc) -> "Power (3ph, Instantaneous)5"/1
  Subsystem10/2(Iabc) -> "Power (3ph, Instantaneous)5"/2
  "Power (3ph, Instantaneous)5"/2 -> Q/1
  "Power (3ph, Instantaneous)5"/1 -> P/1
  connections:
  C/RConn1 -- Subsystem10/LConn3
  c/RConn1 -- Subsystem10/RConn3
  a/RConn1 -- Subsystem10/RConn1
  b/RConn1 -- Subsystem10/RConn2
  B/RConn1 -- Subsystem10/LConn2
  A/RConn1 -- Subsystem10/LConn1

== system inverter_network/Subsystem4 ==
  "Power (3ph, Instantaneous)5" : spsPower3phInstantaneousLib/Power (3ph, Instantaneous)
  Subsystem10 : Subsystem
      settings: PortSchema="{\"entries\":[{\"content\":{\"sides\":[{\"content\":{\"connectorIds\":[\"LConn1\",\"LConn2\",\"LConn3\"]},\"type\":\"ConnectorPlacement.EquallySpacedRectSide\",\"uuid\":\"5e649b81-8d67-47fb-b51d-7fa1d294a0fa\"},{\"content\":{\"connectorIds\":[\"RConn1\",\"RConn2\",\"RConn3\"],\"side\":\"RIGHT\"},\"type\":\"ConnectorPlacement.EquallySpacedRectSide\",\"uuid\":\"b8ce6232-1e24-4620-bb1d-7a04b9b53c9d\"},{\"content\":{\"connectorIds\":[\"Out1\",\"Out2\"],\"side\":\"TOP\"},\"type\":\"ConnectorPlacement.EquallySpacedRectSide\",\"uuid\":\"aabe5581-fbc6-4714-8701-49215a0525de\"}]},\"type\":\"ConnectorPlacement.EquallySpacedConnector\",\"uuid\":\"9c494b08-2ee2-4375-b64d-9899f5cce3ba\"}],\"packageUris\":[\"http://schema.mathworks.com/mf0/Connector/R2020b\"],\"version\":\"1.0\"}"
  A : PMIOPort  Side=Left
  B : PMIOPort  Port=2  Side=Left
  C : PMIOPort  Port=3  Side=Left
  a : PMIOPort  Port=4  Side=Right
  b : PMIOPort  Port=5  Side=Right
  c : PMIOPort  Port=6  Side=Right
  Q : Outport
  P : Outport  Port=2
  wires:
  Subsystem10/1(Vabc) -> "Power (3ph, Instantaneous)5"/1
  Subsystem10/2(Iabc) -> "Power (3ph, Instantaneous)5"/2
  "Power (3ph, Instantaneous)5"/2 -> Q/1
  "Power (3ph, Instantaneous)5"/1 -> P/1
  connections:
  C/RConn1 -- Subsystem10/LConn3
  c/RConn1 -- Subsystem10/RConn3
  a/RConn1 -- Subsystem10/RConn1
  b/RConn1 -- Subsystem10/RConn2
  B/RConn1 -- Subsystem10/LConn2
  A/RConn1 -- Subsystem10/LConn1

== system inverter_network/Subsystem5 ==
  "Power (3ph, Instantaneous)5" : spsPower3phInstantaneousLib/Power (3ph, Instantaneous)
  Subsystem10 : Subsystem
      settings: PortSchema="{\"entries\":[{\"content\":{\"sides\":[{\"content\":{\"connectorIds\":[\"LConn1\",\"LConn2\",\"LConn3\"]},\"type\":\"ConnectorPlacement.EquallySpacedRectSide\",\"uuid\":\"5e649b81-8d67-47fb-b51d-7fa1d294a0fa\"},{\"content\":{\"connectorIds\":[\"RConn1\",\"RConn2\",\"RConn3\"],\"side\":\"RIGHT\"},\"type\":\"ConnectorPlacement.EquallySpacedRectSide\",\"uuid\":\"b8ce6232-1e24-4620-bb1d-7a04b9b53c9d\"},{\"content\":{\"connectorIds\":[\"Out1\",\"Out2\"],\"side\":\"TOP\"},\"type\":\"ConnectorPlacement.EquallySpacedRectSide\",\"uuid\":\"aabe5581-fbc6-4714-8701-49215a0525de\"}]},\"type\":\"ConnectorPlacement.EquallySpacedConnector\",\"uuid\":\"9c494b08-2ee2-4375-b64d-9899f5cce3ba\"}],\"packageUris\":[\"http://schema.mathworks.com/mf0/Connector/R2020b\"],\"version\":\"1.0\"}"
  A : PMIOPort  Side=Left
  B : PMIOPort  Port=2  Side=Left
  C : PMIOPort  Port=3  Side=Left
  a : PMIOPort  Port=4  Side=Right
  b : PMIOPort  Port=5  Side=Right
  c : PMIOPort  Port=6  Side=Right
  P : Outport
  Q : Outport  Port=2
  wires:
  Subsystem10/1(Vabc) -> "Power (3ph, Instantaneous)5"/1
  Subsystem10/2(Iabc) -> "Power (3ph, Instantaneous)5"/2
  "Power (3ph, Instantaneous)5"/2 -> Q/1
  "Power (3ph, Instantaneous)5"/1 -> P/1
  connections:
  C/RConn1 -- Subsystem10/LConn3
  c/RConn1 -- Subsystem10/RConn3
  a/RConn1 -- Subsystem10/RConn1
  b/RConn1 -- Subsystem10/RConn2
  B/RConn1 -- Subsystem10/LConn2
  A/RConn1 -- Subsystem10/LConn1

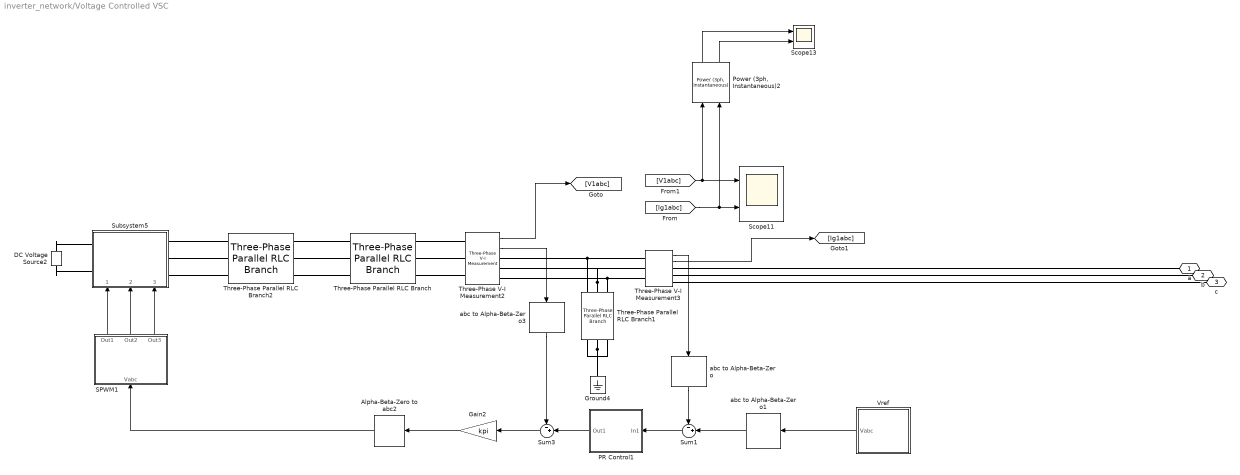
== system inverter_network/Voltage Controlled VSC ==
  Alpha-Beta-Zero to abc2 : spsAlphaBetaZerotoabcLib/Alpha-Beta-Zero to abc
      settings: LibrarySourceBlock=|
      | sps_lib/Control/Alpha-Beta-Zero
      | to abc
  DC Voltage Source2 : spsDCVoltageSourceLib/DC Voltage Source  Amplitude=vdc  Measurements=None
  Gain2 : Gain  Gain=kpi
  Ground4 : spsGroundLib/Ground  LConnTagsString=a
  PR Control1 : Subsystem
  "Power (3ph, Instantaneous)2" : spsPower3phInstantaneousLib/Power (3ph, Instantaneous)
  SPWM1 : Subsystem
  Scope11 : Scope  NumInputPorts=2
  Scope13 : Scope  NumInputPorts=2
  Subsystem5 : Subsystem
      settings: PortSchema="{\"entries\":[{\"content\":{\"sides\":[{\"content\":{\"connectorIds\":[\"LConn1\",\"LConn2\"]},\"type\":\"ConnectorPlacement.EquallySpacedRectSide\",\"uuid\":\"21765539-0567-4900-b052-fb0c809e49e6\"},{\"content\":{\"connectorIds\":[\"RConn1\",\"RConn2\",\"RConn3\"],\"side\":\"RIGHT\"},\"type\":\"ConnectorPlacement.EquallySpacedRectSide\",\"uuid\":\"da60e673-aefd-4ef6-b5b1-e42a137712f7\"},{\"content\":{\"side\":\"TOP\"},\"type\":\"ConnectorPlacement.EquallySpacedRectSide\",\"uuid\":\"b6e664be-1a8c-4c9c-bd73-b93bd6e53381\"},{\"content\":{\"connectorIds\":[\"In1\",\"In2\",\"In3\"],\"side\":\"BOTTOM\"},\"type\":\"ConnectorPlacement.EquallySpacedRectSide\",\"uuid\":\"f785bed7-33ce-41e0-9620-ddd9724794f7\"}]},\"type\":\"ConnectorPlacement.EquallySpacedConnector\",\"uuid\":\"3eaff965-cae1-44ee-8f3f-ae8df46f200b\"}],\"packageUris\":[\"http://schema.mathworks.com/mf0/Connector/R2020b\"],\"version\":\"1.0\"}"
  Sum1 : Sum  Inputs=-+|
  Sum3 : Sum  Inputs=-+|
  Three-Phase Parallel RLC Branch : spsThreePhaseParallelRLCBranchLib/Three-Phase Parallel RLC Branch  LConnTagsString=A|B|C  RConnTagsString=A|B|C  BranchType=L  Resistance=1  Inductance=L_fv  Capacitance=1e-6  Measurements=None
  Three-Phase Parallel RLC Branch1 : spsThreePhaseParallelRLCBranchLib/Three-Phase Parallel RLC Branch  LConnTagsString=A|B|C  RConnTagsString=A|B|C  BranchType=C  Resistance=1  Inductance=vc_l  Capacitance=C_gv  Measurements=None
  Three-Phase Parallel RLC Branch2 : spsThreePhaseParallelRLCBranchLib/Three-Phase Parallel RLC Branch  LConnTagsString=A|B|C  RConnTagsString=A|B|C  BranchType=R  Resistance=0.1  Inductance=L_fv  Capacitance=1e-6  Measurements=None
  Three-Phase V-I Measurement2 : spsThreePhaseVIMeasurementLib/Three-Phase V-I Measurement  VoltageMeasurement=phase-to-ground  SetLabelV=off  LabelV=Vabc  Vpu=off  VpuLL=off  CurrentMeasurement=yes  SetLabelI=off  LabelI=Iabc  Ipu=off  Pbase=100e6  Vbase=500e3  OutputType=Complex  PhasorSimulation=off  PSBequivalent=0
  Three-Phase V-I Measurement3 : spsThreePhaseVIMeasurementLib/Three-Phase V-I Measurement  VoltageMeasurement=phase-to-ground  SetLabelV=off  LabelV=Vabc  Vpu=off  VpuLL=off  CurrentMeasurement=yes  SetLabelI=off  LabelI=Iabc  Ipu=off  Pbase=100e6  Vbase=500e3  OutputType=Complex  PhasorSimulation=off  PSBequivalent=0
  Vref : Subsystem
  abc to Alpha-Beta-Zero : spsabctoAlphaBetaZeroLib/abc to Alpha-Beta-Zero
  abc to Alpha-Beta-Zero1 : spsabctoAlphaBetaZeroLib/abc to Alpha-Beta-Zero
  abc to Alpha-Beta-Zero3 : spsabctoAlphaBetaZeroLib/abc to Alpha-Beta-Zero
  a : PMIOPort  Side=Right
  b : PMIOPort  Port=2  Side=Right
  c : PMIOPort  Port=3  Side=Right
  wires:
  "Power (3ph, Instantaneous)2"/1 -> Scope13/1
  abc to Alpha-Beta-Zero1/1 -> Sum1/2
  abc to Alpha-Beta-Zero3/1 -> Sum3/1
  Three-Phase V-I Measurement2/2 -> abc to Alpha-Beta-Zero3/1
  Sum1/1 -> PR Control1/1(In1)
  SPWM1/2(Out2) -> Subsystem5/2("  2")
  [Ig1abc] -> "Power (3ph, Instantaneous)2"/2, Scope11/2
  abc to Alpha-Beta-Zero/1 -> Sum1/1
  Three-Phase V-I Measurement3/1 -> abc to Alpha-Beta-Zero/1
  SPWM1/1(Out1) -> Subsystem5/1(" 1 ")
  Three-Phase V-I Measurement3/2 -> [Ig1abc]
  "Power (3ph, Instantaneous)2"/2 -> Scope13/2
  [V1abc] -> "Power (3ph, Instantaneous)2"/1, Scope11/1
  PR Control1/1(Out1) -> Sum3/2
  SPWM1/3(Out3) -> Subsystem5/3("  3")
  Gain2/1 -> Alpha-Beta-Zero to abc2/1
  Three-Phase V-I Measurement2/1 -> [V1abc]
  Sum3/1 -> Gain2/1
  Vref/1(Vabc) -> abc to Alpha-Beta-Zero1/1
  Alpha-Beta-Zero to abc2/1 -> SPWM1/1(Vabc)
  connections:
  Three-Phase Parallel RLC Branch1/RConn2 -- Ground4/LConn1 -- Three-Phase Parallel RLC Branch1/RConn1 -- Three-Phase Parallel RLC Branch1/RConn3
  Three-Phase V-I Measurement3/LConn1 -- Three-Phase V-I Measurement2/RConn1 -- Three-Phase Parallel RLC Branch1/LConn1
  Three-Phase Parallel RLC Branch1/LConn2 -- Three-Phase V-I Measurement2/RConn2 -- Three-Phase V-I Measurement3/LConn2
  Three-Phase V-I Measurement3/LConn3 -- Three-Phase V-I Measurement2/RConn3 -- Three-Phase Parallel RLC Branch1/LConn3
  Three-Phase Parallel RLC Branch/RConn1 -- Three-Phase V-I Measurement2/LConn1
  Three-Phase Parallel RLC Branch2/RConn3 -- Three-Phase Parallel RLC Branch/LConn3
  Three-Phase Parallel RLC Branch/RConn2 -- Three-Phase V-I Measurement2/LConn2
  DC Voltage Source2/RConn1 -- Subsystem5/LConn1
  Subsystem5/RConn2 -- Three-Phase Parallel RLC Branch2/LConn2
  DC Voltage Source2/LConn1 -- Subsystem5/LConn2
  Subsystem5/RConn1 -- Three-Phase Parallel RLC Branch2/LConn1
  Three-Phase Parallel RLC Branch/RConn3 -- Three-Phase V-I Measurement2/LConn3
  c/RConn1 -- Three-Phase V-I Measurement3/RConn3
  a/RConn1 -- Three-Phase V-I Measurement3/RConn1
  b/RConn1 -- Three-Phase V-I Measurement3/RConn2
  Subsystem5/RConn3 -- Three-Phase Parallel RLC Branch2/LConn3
  Three-Phase Parallel RLC Branch2/RConn2 -- Three-Phase Parallel RLC Branch/LConn2
  Three-Phase Parallel RLC Branch2/RConn1 -- Three-Phase Parallel RLC Branch/LConn1

== system inverter_network/Current Controlled VSC1/PR Control2 ==
  In1 : Inport
  Constant2 : Constant  Value=0
  Demux3 : Demux  Outputs=3
  Mux4 : Mux  Inputs=3
  Subsystem : Subsystem
  Subsystem1 : Subsystem
  Terminator : Terminator
  Out1 : Outport
  wires:
  Mux4/1 -> Out1/1
  Constant2/1 -> Mux4/3
  In1/1 -> Demux3/1
  Demux3/3 -> Terminator/1
  Demux3/1 -> Subsystem/1(In1)
  Subsystem/1(Out1) -> Mux4/1
  Subsystem1/1(Out1) -> Mux4/2
  Demux3/2 -> Subsystem1/1(In1)

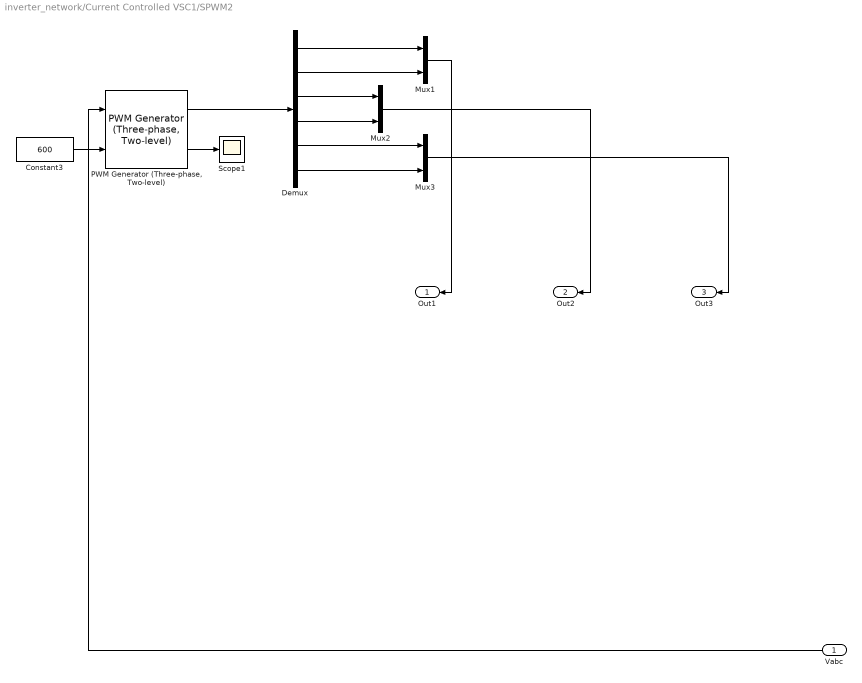
== system inverter_network/Current Controlled VSC1/SPWM2 ==
  Vabc : Inport
  Constant3 : Constant  Value=600
  Demux : Demux  Outputs=6
  Mux1 : Mux  Inputs=2
  Mux2 : Mux  Inputs=2
  Mux3 : Mux  Inputs=2
  "PWM Generator (Three-phase, Two-level)" : eePwmGeneratorTwoLevel/PWM Generator (Three-phase, Two-level)  PWMMode=Continuous PWM (CPWM)  CPWMMode=SPWM: sinusoidal PWM  DPWMMode=60 DPWM: 60 degree discontinuous PWM  fsw=10000  Ts=1/(100*10000)
      settings: LibrarySourceBlock=|
      | ee_sl_lib/Pulse Width
      | Modulation/PWM Generator
      | (Three-phase, Two-level)
  Scope1 : Scope
  Out1 : Outport
  Out2 : Outport  Port=2
  Out3 : Outport  Port=3
  wires:
  "PWM Generator (Three-phase, Two-level)"/2 -> Scope1/1
  Demux/2 -> Mux1/2
  Vabc/1 -> "PWM Generator (Three-phase, Two-level)"/1
  Demux/6 -> Mux3/2
  Demux/1 -> Mux1/1
  Constant3/1 -> "PWM Generator (Three-phase, Two-level)"/2
  Mux2/1 -> Out2/1
  Demux/4 -> Mux2/2
  "PWM Generator (Three-phase, Two-level)"/1 -> Demux/1
  Demux/3 -> Mux2/1
  Demux/5 -> Mux3/1
  Mux1/1 -> Out1/1
  Mux3/1 -> Out3/1

== system inverter_network/Current Controlled VSC1/Subsystem ==
  In1 : Inport
  Constant5 : Constant  Value=vref_rms
  Divide1 : Product  Inputs=*/
  Gain2 : Gain  Gain=3
  Gain3 : Gain  Gain=975/400
  Out1 : Outport
  wires:
  Gain3/1 -> Divide1/1
  Constant5/1 -> Gain2/1
  Gain2/1 -> Divide1/2
  In1/1 -> Gain3/1
  Divide1/1 -> Out1/1

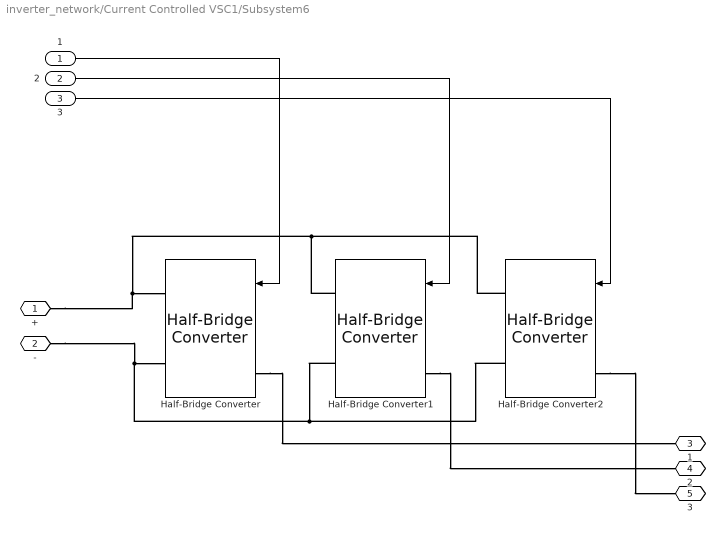
== system inverter_network/Current Controlled VSC1/Subsystem6 ==
  " 1 " : Inport
  "  2" : Inport  Port=2
  "  3" : Inport  Port=3
  Half-Bridge Converter : spsHalfBridgeConverterLib/Half-Bridge Converter  ModelType=Switching devices  Ron=1e-3  Rs=1e6  Cs=inf  Vforward=[0,0]  Ron_Diode=1e-3  Rs_Diode=1e6  Cs_Diode=inf  Vf_Diode=1e-3  Rs_CurrentSource=inf  Ron_ACsource=1e-3
      settings: LibrarySourceBlock=sps_lib/Power Electronics/Half-Bridge Converter
  Half-Bridge Converter1 : spsHalfBridgeConverterLib/Half-Bridge Converter  ModelType=Switching devices  Ron=1e-3  Rs=1e6  Cs=inf  Vforward=[0,0]  Ron_Diode=1e-3  Rs_Diode=1e6  Cs_Diode=inf  Vf_Diode=1e-3  Rs_CurrentSource=inf  Ron_ACsource=1e-3
      settings: LibrarySourceBlock=sps_lib/Power Electronics/Half-Bridge Converter
  Half-Bridge Converter2 : spsHalfBridgeConverterLib/Half-Bridge Converter  ModelType=Switching devices  Ron=1e-3  Rs=1e6  Cs=inf  Vforward=[0,0]  Ron_Diode=1e-3  Rs_Diode=1e6  Cs_Diode=inf  Vf_Diode=1e-3  Rs_CurrentSource=inf  Ron_ACsource=1e-3
      settings: LibrarySourceBlock=sps_lib/Power Electronics/Half-Bridge Converter
  + : PMIOPort  Side=Left
  - : PMIOPort  Port=2  Side=Left
  1 : PMIOPort  Port=3  Side=Right
  2 : PMIOPort  Port=4  Side=Right
  3 : PMIOPort  Port=5  Side=Right
  wires:
  "  2"/1 -> Half-Bridge Converter1/1
  "  3"/1 -> Half-Bridge Converter2/1
  " 1 "/1 -> Half-Bridge Converter/1
  connections:
  Half-Bridge Converter/LConn1 -- 1/RConn1
  Half-Bridge Converter2/RConn1 -- Half-Bridge Converter1/RConn1 -- Half-Bridge Converter/RConn1 -- +/RConn1
  Half-Bridge Converter2/RConn2 -- Half-Bridge Converter1/RConn2 -- Half-Bridge Converter/RConn2 -- -/RConn1
  Half-Bridge Converter2/LConn1 -- 3/RConn1
  Half-Bridge Converter1/LConn1 -- 2/RConn1

== system inverter_network/Current Controlled VSC1/Subsystem7 ==
  Three-Phase V-I Measurement2 : spsThreePhaseVIMeasurementLib/Three-Phase V-I Measurement  VoltageMeasurement=phase-to-ground  SetLabelV=off  LabelV=Vabc  Vpu=off  VpuLL=off  CurrentMeasurement=yes  SetLabelI=off  LabelI=Iabc  Ipu=off  Pbase=100e6  Vbase=500e3  OutputType=Complex  PhasorSimulation=off  PSBequivalent=0
  A : PMIOPort  Side=Left
  B : PMIOPort  Port=2  Side=Left
  C : PMIOPort  Port=3  Side=Left
  a : PMIOPort  Port=4  Side=Right
  b : PMIOPort  Port=5  Side=Right
  c : PMIOPort  Port=6  Side=Right
  Iabc : Outport
  wires:
  Three-Phase V-I Measurement2/2 -> Iabc/1
  connections:
  Three-Phase V-I Measurement2/LConn1 -- A/RConn1
  Three-Phase V-I Measurement2/RConn3 -- c/RConn1
  Three-Phase V-I Measurement2/RConn1 -- a/RConn1
  Three-Phase V-I Measurement2/LConn2 -- B/RConn1
  Three-Phase V-I Measurement2/RConn2 -- b/RConn1
  Three-Phase V-I Measurement2/LConn3 -- C/RConn1

== system inverter_network/Current Controlled VSC1/Subsystem8 ==
  Three-Phase V-I Measurement3 : spsThreePhaseVIMeasurementLib/Three-Phase V-I Measurement  VoltageMeasurement=phase-to-ground  SetLabelV=off  LabelV=Vabc  Vpu=off  VpuLL=off  CurrentMeasurement=yes  SetLabelI=off  LabelI=Iabc  Ipu=off  Pbase=100e6  Vbase=500e3  OutputType=Complex  PhasorSimulation=off  PSBequivalent=0
  A : PMIOPort  Side=Left
  B : PMIOPort  Port=2  Side=Left
  C : PMIOPort  Port=3  Side=Left
  Vabc : Outport
  wires:
  Three-Phase V-I Measurement3/1 -> Vabc/1
  connections:
  Three-Phase V-I Measurement3/LConn1 -- A/RConn1
  Three-Phase V-I Measurement3/LConn2 -- B/RConn1
  Three-Phase V-I Measurement3/LConn3 -- C/RConn1

== system inverter_network/Current Controlled VSC1/Subsystem9 ==
  Three-Phase V-I Measurement : spsThreePhaseVIMeasurementLib/Three-Phase V-I Measurement  VoltageMeasurement=phase-to-ground  SetLabelV=off  LabelV=Vabc  Vpu=off  VpuLL=off  CurrentMeasurement=yes  SetLabelI=off  LabelI=Iabc  Ipu=off  Pbase=100e6  Vbase=500e3  OutputType=Complex  PhasorSimulation=off  PSBequivalent=0
  A : PMIOPort  Side=Left
  B : PMIOPort  Port=2  Side=Left
  C : PMIOPort  Port=3  Side=Left
  a : PMIOPort  Port=4  Side=Right
  b : PMIOPort  Port=5  Side=Right
  c : PMIOPort  Port=6  Side=Right
  Vabc : Outport
  Iabc : Outport  Port=2
  wires:
  Three-Phase V-I Measurement/2 -> Iabc/1
  Three-Phase V-I Measurement/1 -> Vabc/1
  connections:
  Three-Phase V-I Measurement/RConn1 -- a/RConn1
  Three-Phase V-I Measurement/LConn2 -- B/RConn1
  Three-Phase V-I Measurement/RConn3 -- c/RConn1
  Three-Phase V-I Measurement/LConn1 -- A/RConn1
  Three-Phase V-I Measurement/LConn3 -- C/RConn1
  Three-Phase V-I Measurement/RConn2 -- b/RConn1

== system inverter_network/Current Controlled VSC1/dq0 to Alpha Beta1 ==
  dq0 : Inport
  wt : Inport  Port=2
  dq0 to Alpha-Beta-Zero : spsdq0toAlphaBetaZeroLib/dq0 to Alpha-Beta-Zero  Alignment=90 degrees behind phase A axis
  al_be_0 : Outport
  wires:
  dq0 to Alpha-Beta-Zero/1 -> al_be_0/1
  wt/1 -> dq0 to Alpha-Beta-Zero/2
  dq0/1 -> dq0 to Alpha-Beta-Zero/1

== system inverter_network/Current Controlled VSC2/PR Control2 ==
  In1 : Inport
  Constant2 : Constant  Value=0
  Demux3 : Demux  Outputs=3
  Mux4 : Mux  Inputs=3
  Subsystem : Subsystem
  Subsystem1 : Subsystem
  Terminator : Terminator
  Out1 : Outport
  wires:
  Mux4/1 -> Out1/1
  Constant2/1 -> Mux4/3
  In1/1 -> Demux3/1
  Demux3/3 -> Terminator/1
  Demux3/1 -> Subsystem/1(In1)
  Subsystem/1(Out1) -> Mux4/1
  Subsystem1/1(Out1) -> Mux4/2
  Demux3/2 -> Subsystem1/1(In1)

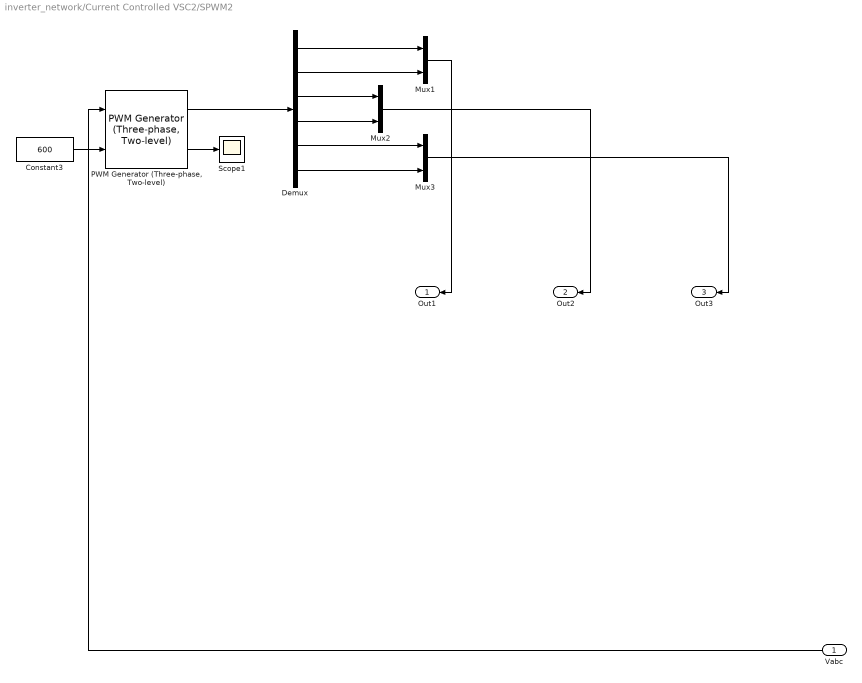
== system inverter_network/Current Controlled VSC2/SPWM2 ==
  Vabc : Inport
  Constant3 : Constant  Value=600
  Demux : Demux  Outputs=6
  Mux1 : Mux  Inputs=2
  Mux2 : Mux  Inputs=2
  Mux3 : Mux  Inputs=2
  "PWM Generator (Three-phase, Two-level)" : eePwmGeneratorTwoLevel/PWM Generator (Three-phase, Two-level)  PWMMode=Continuous PWM (CPWM)  CPWMMode=SPWM: sinusoidal PWM  DPWMMode=60 DPWM: 60 degree discontinuous PWM  fsw=10000  Ts=1/(100*10000)
      settings: LibrarySourceBlock=|
      | ee_sl_lib/Pulse Width
      | Modulation/PWM Generator
      | (Three-phase, Two-level)
  Scope1 : Scope
  Out1 : Outport
  Out2 : Outport  Port=2
  Out3 : Outport  Port=3
  wires:
  "PWM Generator (Three-phase, Two-level)"/2 -> Scope1/1
  Demux/2 -> Mux1/2
  Vabc/1 -> "PWM Generator (Three-phase, Two-level)"/1
  Demux/6 -> Mux3/2
  Demux/1 -> Mux1/1
  Constant3/1 -> "PWM Generator (Three-phase, Two-level)"/2
  Mux2/1 -> Out2/1
  Demux/4 -> Mux2/2
  "PWM Generator (Three-phase, Two-level)"/1 -> Demux/1
  Demux/3 -> Mux2/1
  Demux/5 -> Mux3/1
  Mux1/1 -> Out1/1
  Mux3/1 -> Out3/1

== system inverter_network/Current Controlled VSC2/Subsystem ==
  In1 : Inport
  Constant5 : Constant  Value=vref_rms
  Divide1 : Product  Inputs=*/
  Gain2 : Gain  Gain=3
  Gain3 : Gain  Gain=975/400
  Out1 : Outport
  wires:
  Gain3/1 -> Divide1/1
  Constant5/1 -> Gain2/1
  Gain2/1 -> Divide1/2
  In1/1 -> Gain3/1
  Divide1/1 -> Out1/1

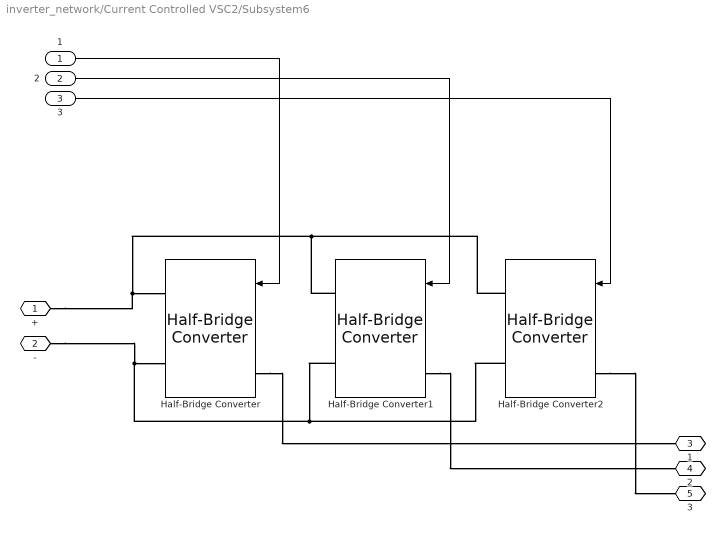
== system inverter_network/Current Controlled VSC2/Subsystem6 ==
  " 1 " : Inport
  "  2" : Inport  Port=2
  "  3" : Inport  Port=3
  Half-Bridge Converter : spsHalfBridgeConverterLib/Half-Bridge Converter  ModelType=Switching devices  Ron=1e-3  Rs=1e6  Cs=inf  Vforward=[0,0]  Ron_Diode=1e-3  Rs_Diode=1e6  Cs_Diode=inf  Vf_Diode=1e-3  Rs_CurrentSource=inf  Ron_ACsource=1e-3
      settings: LibrarySourceBlock=sps_lib/Power Electronics/Half-Bridge Converter
  Half-Bridge Converter1 : spsHalfBridgeConverterLib/Half-Bridge Converter  ModelType=Switching devices  Ron=1e-3  Rs=1e6  Cs=inf  Vforward=[0,0]  Ron_Diode=1e-3  Rs_Diode=1e6  Cs_Diode=inf  Vf_Diode=1e-3  Rs_CurrentSource=inf  Ron_ACsource=1e-3
      settings: LibrarySourceBlock=sps_lib/Power Electronics/Half-Bridge Converter
  Half-Bridge Converter2 : spsHalfBridgeConverterLib/Half-Bridge Converter  ModelType=Switching devices  Ron=1e-3  Rs=1e6  Cs=inf  Vforward=[0,0]  Ron_Diode=1e-3  Rs_Diode=1e6  Cs_Diode=inf  Vf_Diode=1e-3  Rs_CurrentSource=inf  Ron_ACsource=1e-3
      settings: LibrarySourceBlock=sps_lib/Power Electronics/Half-Bridge Converter
  + : PMIOPort  Side=Left
  - : PMIOPort  Port=2  Side=Left
  1 : PMIOPort  Port=3  Side=Right
  2 : PMIOPort  Port=4  Side=Right
  3 : PMIOPort  Port=5  Side=Right
  wires:
  "  2"/1 -> Half-Bridge Converter1/1
  "  3"/1 -> Half-Bridge Converter2/1
  " 1 "/1 -> Half-Bridge Converter/1
  connections:
  Half-Bridge Converter/LConn1 -- 1/RConn1
  Half-Bridge Converter2/RConn1 -- Half-Bridge Converter1/RConn1 -- Half-Bridge Converter/RConn1 -- +/RConn1
  Half-Bridge Converter2/RConn2 -- Half-Bridge Converter1/RConn2 -- Half-Bridge Converter/RConn2 -- -/RConn1
  Half-Bridge Converter2/LConn1 -- 3/RConn1
  Half-Bridge Converter1/LConn1 -- 2/RConn1
